simulink model "Reductor"  (R2015a)
settings: Solver=ode45  StartTime=0.0  StopTime=0.02  RelTol=1e-3
values from neighbouring files (symbols this model uses):
  C = 120e-6    (= 0.00012)    [Reductor_code.m]
  D = 0.5    [Reductor_code.m]
  L = 470e-6    (= 0.00047)    [Reductor_code.m]
  R = 100    [Reductor_code.m]
  Vd = 12    [Reductor_code.m]
libraries: powerlib x12, powerlib_meascontrol x2
settings Model: Creator=Daymee  LastModifiedBy=Daymee

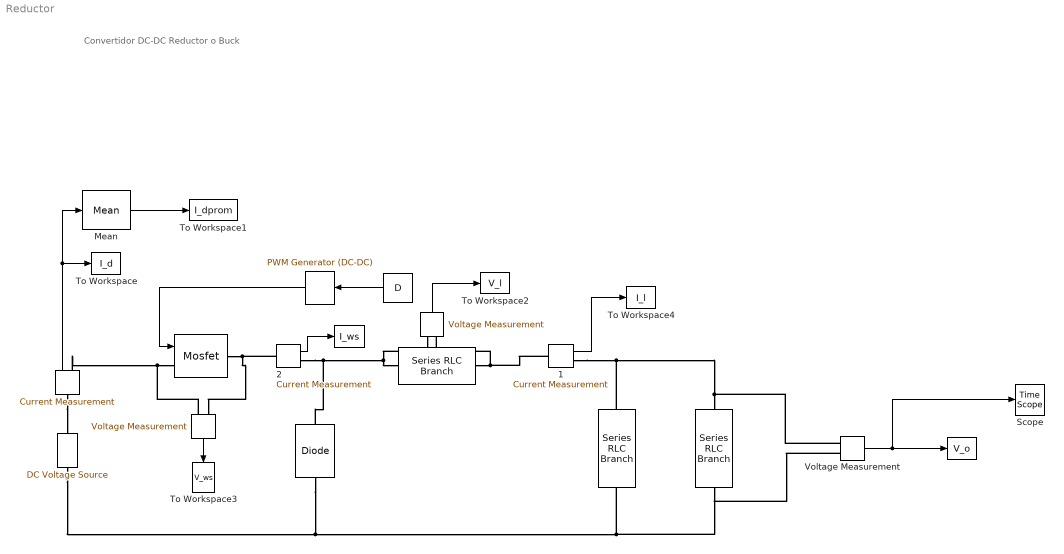
== system Reductor ==
  note: Convertidor DC-DC Reductor o Buck
  " " : powerlib/Measurements/Current Measurement  PhasorSimulation=off  OutputType=Complex  PSBequivalent=0
  " 1" : powerlib/Measurements/Current Measurement  PhasorSimulation=off  OutputType=Complex  PSBequivalent=0
  " 2" : powerlib/Measurements/Current Measurement  PhasorSimulation=off  OutputType=Complex  PSBequivalent=0
  " " : powerlib/Measurements/Voltage Measurement  PhasorSimulation=off  OutputType=Complex  PSBequivalent=0
  " " : powerlib/Power Electronics/Diode  Ron=0.001  Lon=0  Vf=0.8  IC=0  UseSnubber=off  Rs=500  Cs=250e-9  Measurements=off
  "  " : powerlib/Elements/Series RLC Branch  LConnTagsString=__new0  RConnTagsString=__new0  BranchType=L  Resistance=1  Inductance=L  SetiL0=off  InitialCurrent=0  Capacitance=1e-6  Setx0=off  InitialVoltage=0  Measurements=None
  "   " : powerlib/Elements/Series RLC Branch  LConnTagsString=__new0  RConnTagsString=__new0  BranchType=C  Resistance=1  Inductance=1e-3  SetiL0=off  InitialCurrent=0  Capacitance=C  Setx0=off  InitialVoltage=0  Measurements=None
  "     " : powerlib/Elements/Series RLC Branch  LConnTagsString=__new0  RConnTagsString=__new0  BranchType=R  Resistance=R  Inductance=1e-3  SetiL0=off  InitialCurrent=0  Capacitance=C  Setx0=off  InitialVoltage=0  Measurements=None
  "       " : powerlib/Electrical Sources/DC Voltage Source  Amplitude=Vd  Measurements=None
  " " : powerlib_meascontrol/Pulse & Signal Generators/PWM Generator (DC-DC)  Fsw=Fs  Ts=0
  "         " : powerlib/Power Electronics/Mosfet  Ron=0.1  Lon=0  Rd=0.01  Vfd=0  IC=0  Rs=1e5  Cs=inf  Measurements=off
  "               " : Constant  Value=D
  " " : ToWorkspace  VariableName=I_ws  SampleTime=-1
  "                     " : ToWorkspace  VariableName=V_o  SampleTime=-1
  " " : powerlib/Measurements/Voltage Measurement  PhasorSimulation=off  OutputType=Complex  PSBequivalent=0
  Mean : powerlib_meascontrol/Measurements/Mean  Freq=Fs  Vinit=0  Ts=0
  Scope : TimeScope
  To Workspace : ToWorkspace  VariableName=I_d  SampleTime=-1
  To Workspace1 : ToWorkspace  VariableName=I_dprom  SampleTime=-1
  To Workspace2 : ToWorkspace  VariableName=V_l  SampleTime=-1
  To Workspace3 : ToWorkspace  VariableName=V_ws  SampleTime=-1
  To Workspace4 : ToWorkspace  VariableName=I_l  SampleTime=-1
  Voltage Measurement : powerlib/Measurements/Voltage Measurement  PhasorSimulation=off  OutputType=Complex  PSBequivalent=0
  wires:
  " "/1 -> Mean/1, To Workspace/1
  Mean/1 -> To Workspace1/1
  " "/1 -> "         "/1
  "               "/1 -> " "/1
  Voltage Measurement/1 -> Scope/1, "                     "/1
  " "/1 -> To Workspace2/1
  " "/1 -> To Workspace3/1
  " 1"/1 -> To Workspace4/1
  " 2"/1 -> " "/1
  connections:
  " "/RConn1 -- " 2"/RConn1 -- "  "/LConn1 -- " "/LConn1
  "   "/LConn1 -- Voltage Measurement/LConn1 -- "     "/LConn1 -- " 1"/RConn1
  "       "/LConn1 -- " "/LConn1 -- Voltage Measurement/LConn2 -- "     "/RConn1 -- "   "/RConn1
  " "/LConn1 -- "       "/RConn1
  " "/RConn1 -- " "/LConn2 -- "         "/LConn1
  "  "/RConn1 -- " 1"/LConn1 -- " "/LConn2
  "         "/RConn1 -- " 2"/LConn1 -- " "/LConn1
